simulink model "FMReceiverSimulinkExample"  (R2016b)
settings: Solver=FixedStepDiscrete  StartTime=0.0  StopTime=inf  RelTol=1e-3
PreLoadFcn:
  | fmRxParams = helperFMConfig;
InitFcn:
  | fmRxParams = helperFMConfig;
libraries: simulink x2, dspsnks4 x1, commsource2 x1, commanabbnd3 x1, commblksprivate x1, sdrrlib x1
Description:
  | This model uses Universal Software Radio Peripheral (USRP) hardware with Simulink(R) to perform FM demodulation and stereo decoding.
settings Model: Creator=The MathWorks, Inc.  LastModifiedBy=Eduardo
settings DataIOCC: SaveFormat=Structure  SaveOutput=off  SignalLogging=off  DSMLogging=off  SaveTime=off
settings OptimizationCC: ExpressionDepthLimit=2147483647  EfficientMapNaN2IntZero=off  LifeSpan=inf  SimCompilerOptimization=on
settings DebuggingCC: UnderspecifiedInitializationDetection=Classic  MergeDetectMultiDrivingBlocksExec=none  SolverPrmCheckMsg=warning  InheritedTsInSrcMsg=none  MultiTaskCondExecSysMsg=none  ParameterPrecisionLossMsg=none  FcnCallInpInsideContextMsg=warning  AllowSymbolicDim=off  StateNameClashWarn=warning  SFUnexpectedBacktrackingDiag=warning  SFNoUnconditionalDefaultTransitionDiag=warning  SFExecutionAtInitializationDiag=none
settings HardwareCC: ProdBitPerPointer=32  ProdBitPerSizeT=32  ProdBitPerPtrDiffT=32  ProdLargestAtomicFloat=None  ProdIntDivRoundTo=Undefined  ProdEndianess=Unspecified  ProdWordSize=32  ProdHWDeviceType=32-bit Generic  TargetBitPerPointer=64  TargetBitPerSizeT=64  TargetBitPerPtrDiffT=64  TargetLongLongMode=on  TargetIntDivRoundTo=Zero  TargetEndianess=LittleEndian  TargetWordSize=64  TargetHWDeviceType=Generic->MATLAB Host Computer  ProdEqTarget=off
settings ModelReferenceCC: PropagateSignalLabelsOutOfModel=off
settings SFSimCC: SimIntegrity=off
settings RTWCC: CustomSourceCode=|
  | #include <stdio.h>
  | #include <stdlib.h>
settings CodeAppCC: MaxIdLength=128
settings GRTTargetCC: TargetLangStandard=C89/C90 (ANSI)  GeneratePreprocessorConditionals=Disable all  CombineOutputUpdateFcns=off  GRTInterface=on
settings ConfigComp: CovMetricSettings=dw  CovHtmlReporting=on  CovSaveCumulativeToWorkspaceVar=on  CovSaveSingleToWorkspaceVar=on  CovExternalEMLEnable=off  CovSFcnEnable=off

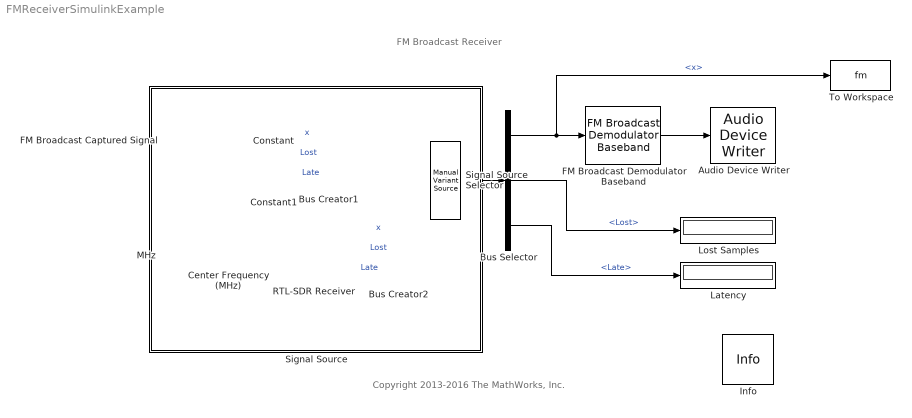
== system FMReceiverSimulinkExample ==
  note: Copyright 2013-2016 The MathWorks, Inc.
  note: FM Broadcast Receiver
  Audio Device Writer : dspsnks4/Audio Device Writer  Driver=DirectSound  Device=Default  InheritSampleRate=on  SampleRate=44100  BitDepth=16-bit integer  BufferSize=4096  NumBuffers=10  DefaultOutputChannelMapping=on  OutputChannelMapping=1:2  OutputNumUnderrunSamples=off  DriverIdx=1  DeviceWarnFlag=''
  Bus Creator1 : BusCreator  Inputs=3
  Bus Creator2 : BusCreator  Inputs=3
  Bus Selector : BusSelector  OutputSignals=x,Lost,Late
  Center Frequency (MHz) : simulink/Math Operations/Slider Gain  low=87.9  gain=90.5  high=107.9
  Constant : Constant  Value=0
  Constant1 : Constant
  FM Broadcast Captured Signal : commsource2/Baseband File Reader  Filename=fm_capture_01.bb  InheritSampleTimeFromFile=on  SampleTime=1  SamplesPerFrame=fmRxParams.FrontEndSamplesPerFrame  CyclicRepetition=on  FileEndOutputPort=off  SimulateUsing=Code generation
  FM Broadcast Demodulator Baseband : commanabbnd3/FM Broadcast Demodulator Baseband  SampleRate=fmRxParams.FrontEndSampleRate  FrequencyDeviation=fmRxParams.FrequencyDeviation  FilterTimeConstant=fmRxParams.FilterTimeConstant  AudioSampleRate=fmRxParams.AudioSampleRate  PlaySound=off  BufferSize=fmRxParams.BufferSize  Stereo=on  SimulateUsing=Code generation
  Info : commblksprivate/Info  SystemSampleTime=-1
  Latency : Display
  Lost Samples : Display
  MHz : Constant  Value=1e6  VectorParams1D=off  SampleTime=-1  FramePeriod=-1
  RTL-SDR Receiver : sdrrlib/RTL-SDR Receiver  SourceLibraryInfo="This block requires <a href=\"http://www.mathworks.com/hardware-support/rtl-sdr.html\">Communications System Toolbox Support Package for RTL-SDR Radio</a>"  sobjType=sdrr.internal.SDRRTLReceiverSL  IPAddress=0  dataUDPPort=-1  ctrlUDPPort=-1  subDeviceList=nosubdev  sdrBlockType=SDRBlockTypeSLT.SDRRxBlock  requester=UNUSED_BY_SFCN  sdrExecutionMode=SDRExecutionModeSLT.ExecModeHW  LostSamplesOutputPort=on  OutputDataType=single  FrameLength=fmRxParams.FrontEndSamplesPerFrame  EnableBurstMode=off  NumFramesInBurst=20  BypassUserLogic=off  DecimatorSelect=DDC decimator  SourceSelect=RF data  SineAmplitude=16000  EnableInternalClock=off  BypassIQBalance=off  CenterFrequency=102.5e6  IFBandwidth=40e6  ADCRateSource=Dialog  ADCRate=fmRxParams.FrontEndSampleRate  CenterFrequencySource=Input port  GainSource=AGC  IntermediateFrequency=0  Gain=0  DecimationFactorSource=Dialog  DecimationFactor=512  RFFrequencyIsTunable=logical(1)  SampleTime=(fmRxParams.FrontEndSamplesPerFrame)/(fmRxParams.FrontEndSampleRate)  IFBandwidthSource=Dialog  SineFrequency=30000  BypassDCBlockingFilter=off  IntermediateFrequencySource=Dialog  IQBalanceCoefficients=64  SkipAllHardwareResetAndInitialization=off  EnableIQCalibrationTable=on  CacheIQCalibrationTable=off  EnableOffsetTuning=off  EnableRTLAGC=off  EnableTestMode=off  EnableTunerAGC=on  FrequencyCorrectionSource=Dialog  FrequencyCorrection=0  NumMLBuffers=128  NumUSBBuffers=16  LatencyOutputPort=on  RTLCrystalFrequency=28800000  TunerCrystalFrequency=28800000
  Signal Source : Subsystem
      mask Display: disp('')
  Signal Source Selector : simulink/Signal Routing/Manual Variant Source  NumChoices=2  OverrideUsingVariant=V_2
  To Workspace : ToWorkspace  VariableName=fm  SampleTime=-1
      settings: Save2DSignal=2-D array (concatenate along first dimension)
  wires:
  MHz/1 -> Center Frequency (MHz)/1
  Center Frequency (MHz)/1 -> RTL-SDR Receiver/1
  FM Broadcast Demodulator Baseband/1 -> Audio Device Writer/1
  FM Broadcast Captured Signal/1 -> Bus Creator1/1  "x"
  Constant/1 -> Bus Creator1/2  "Lost"
  Constant1/1 -> Bus Creator1/3  "Late"
  Bus Creator1/1 -> Signal Source Selector/1
  RTL-SDR Receiver/1 -> Bus Creator2/1  "x"
  RTL-SDR Receiver/2 -> Bus Creator2/2  "Lost"
  RTL-SDR Receiver/3 -> Bus Creator2/3  "Late"
  Bus Creator2/1 -> Signal Source Selector/2
  Signal Source Selector/1 -> Bus Selector/1
  Bus Selector/1 -> To Workspace/1, FM Broadcast Demodulator Baseband/1  "<x>"
  Bus Selector/2 -> Lost Samples/1  "<Lost>"
  Bus Selector/3 -> Latency/1  "<Late>"

== system FMReceiverSimulinkExample/Signal Source ==
